simulink model "Blocos"  (R2022a)
settings: Solver=ode8  StartTime=0.0  StopTime=inf  FixedStep=0.01  RelTol=1e-3  EnableMultiTasking=on
libraries: dspstat3 x3
settings Model: Creator=MSI  LastModifiedBy=MSI
settings SolverCC: PositivePriorityOrder=on
settings OptimizationCC: EnhancedBackFolding=on  PassReuseOutputArgsAs=Individual arguments  ZeroExternalMemoryAtStartup=off  ZeroInternalMemoryAtStartup=off  MaxStackSize=64  OptimizeBlockOrder=speed  DifferentSizesBufferReuse=on  OptimizationCustomize=off  EfficientTunableParamExpr=on
settings DebuggingCC: ParameterTunabilityLossMsg=error
settings HardwareCC: ProdBitPerPointer=32  ProdBitPerSizeT=32  ProdBitPerPtrDiffT=32  ProdLargestAtomicInteger=Long  ProdLargestAtomicFloat=Double  ProdWordSize=32  ProdLongLongMode=on  ProdHWDeviceType=ARM Compatible->ARM Cortex
settings RTWCC: SystemTargetFile=ert.tlc  HardwareBoard=Raspberry Pi  TLCOptions="-aInlineSetEventsForThisBaseRateFcn=TLC_FALSE -aSuppressMultiTaskScheduler=TLC_FALSE  -aRateBasedStepFcn=0"  TemplateMakefile=ert_default_tmf  Toolchain=GNU GCC Embedded Linux  BuildConfiguration=Faster Runs
settings CodeAppCC: ForceParamTrailComments=on  IgnoreCustomStorageClasses=off  OperatorAnnotations=on  SimulinkDataObjDesc=on  SFDataObjDesc=on  InsertBlockDesc=on
settings ERTTargetCC: SupportVariableSizeSignals=on  ExtModeTransport=2  ExtModeStaticAlloc=on  ExtModeMexFile=ext_xcp  ExtModeIntrfLevel=Level2 - Open

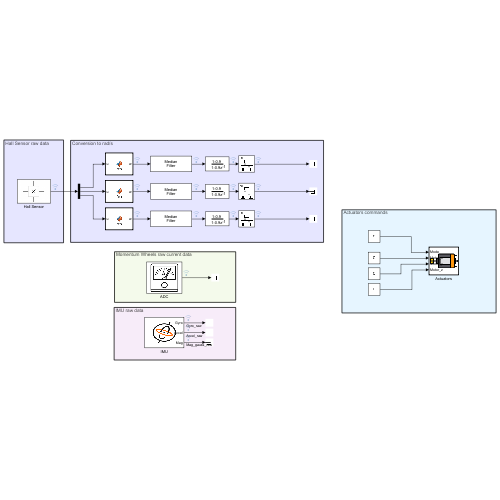
[thumbnail: Simulink's stored preview of the top-level diagram]
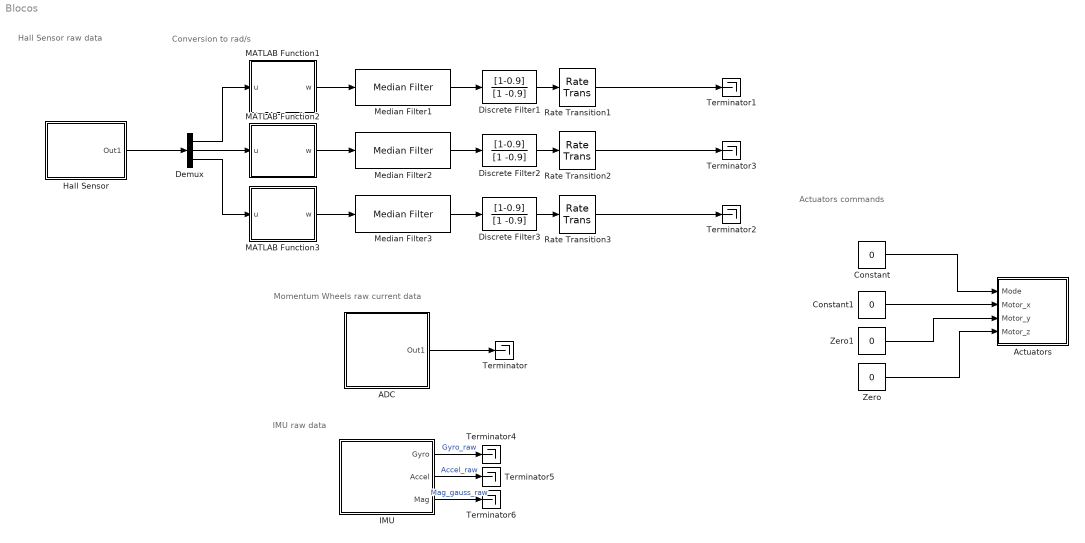
== system Blocos ==
  note: Actuators commands
  note: IMU raw data
  note: Momentum Wheels raw current data
  note: Hall Sensor raw data
  note: Conversion to rad/s
  ADC : Subsystem
      mask Display: image('$imagefile'); % Use "Edit Image" on toolstrip to change.
  Actuators : Subsystem  TreatAsAtomicUnit=on  SystemSampleTime=0.01
      mask Display: image('$imagefile'); % Use "Edit Image" on toolstrip to change.
  Constant : Constant  Value=0
  Constant1 : Constant  Value=0
  Demux : Demux  Outputs=3
  Discrete Filter1 : DiscreteFilter  Numerator=[1-0.9]  Denominator=[1 -0.9]  SampleTime=0.01
  Discrete Filter2 : DiscreteFilter  Numerator=[1-0.9]  Denominator=[1 -0.9]  SampleTime=0.01
  Discrete Filter3 : DiscreteFilter  Numerator=[1-0.9]  Denominator=[1 -0.9]  SampleTime=0.01
  Hall Sensor : Subsystem
      mask Display: image('$imagefile'); % Use "Edit Image" on toolstrip to change.
  IMU : Subsystem
      mask Display: image('$imagefile'); % Use "Edit Image" on toolstrip to change.
  MATLAB Function1 : MATLAB Function  TreatAsAtomicUnit=on
  MATLAB Function2 : MATLAB Function  TreatAsAtomicUnit=on
  MATLAB Function3 : MATLAB Function  TreatAsAtomicUnit=on
  Median Filter1 : dspstat3/Median Filter  WindowLength=5  SimulateUsing=Interpreted execution
      settings: SourceProductBaseCode=DS
  Median Filter2 : dspstat3/Median Filter  WindowLength=5  SimulateUsing=Interpreted execution
      settings: SourceProductBaseCode=DS
  Median Filter3 : dspstat3/Median Filter  WindowLength=5  SimulateUsing=Interpreted execution
      settings: SourceProductBaseCode=DS
  Rate Transition1 : RateTransition
  Rate Transition2 : RateTransition
  Rate Transition3 : RateTransition
  Terminator{,1..6} (7 alike) : Terminator
  Zero : Constant  Value=0  OutDataTypeStr=Inherit: Inherit via back propagation
  Zero1 : Constant  Value=0  OutDataTypeStr=Inherit: Inherit via back propagation
  wires:
  Constant/1 -> Actuators/1(Mode)
  Constant1/1 -> Actuators/2(Motor_x)
  Zero/1 -> Actuators/4(Motor_z)
  Zero1/1 -> Actuators/3(Motor_y)
  IMU/1(Gyro) -> Terminator4/1  "Gyro_raw"
  IMU/2(Accel) -> Terminator5/1  "Accel_raw"
  IMU/3(Mag) -> Terminator6/1  "Mag_gauss_raw"
  MATLAB Function3/1(w) -> Median Filter3/1
  MATLAB Function2/1(w) -> Median Filter2/1
  MATLAB Function1/1(w) -> Median Filter1/1
  Demux/2 -> MATLAB Function2/1(u)
  Demux/1 -> MATLAB Function1/1(u)
  Demux/3 -> MATLAB Function3/1(u)
  Discrete Filter3/1 -> Rate Transition3/1
  Rate Transition3/1 -> Terminator2/1
  Median Filter3/1 -> Discrete Filter3/1
  Rate Transition1/1 -> Terminator1/1
  Median Filter1/1 -> Discrete Filter1/1
  Discrete Filter1/1 -> Rate Transition1/1
  Rate Transition2/1 -> Terminator3/1
  Median Filter2/1 -> Discrete Filter2/1
  Discrete Filter2/1 -> Rate Transition2/1
  Hall Sensor/1(Out1) -> Demux/1
  ADC/1(Out1) -> Terminator/1

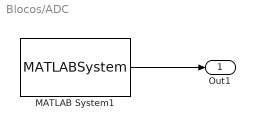
== system Blocos/ADC ==
  MATLAB System1 : MATLABSystem  System=read_current  SampleTime=0.01
      mask Type: read_current
      mask Display:
      | disp('ADC');
      | port_label('output',1,'current');
  Out1 : Outport
  wires:
  MATLAB System1/1 -> Out1/1

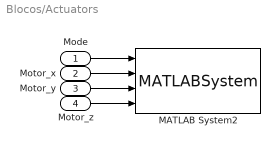
== system Blocos/Actuators ==
  Mode : Inport
  Motor_x : Inport  Port=2
  Motor_y : Inport  Port=3
  Motor_z : Inport  Port=4
  MATLAB System2 : MATLABSystem  System=arduinoPwmWrite
      mask Type: arduinoPwmWrite
      mask Display:
      | disp('PWM INO');
      | port_label('input',1,'mode');
      | port_label('input',2,'pwm_0');
      | port_label('input',3,'pwm_1');
      | port_label('input',4,'pwm_2');
  wires:
  Motor_y/1 -> MATLAB System2/3
  Motor_x/1 -> MATLAB System2/2
  Motor_z/1 -> MATLAB System2/4
  Mode/1 -> MATLAB System2/1

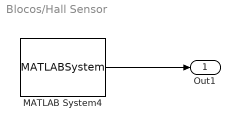
== system Blocos/Hall Sensor ==
  MATLAB System4 : MATLABSystem  System=read_n_crossings  SampleTime=0.01
      mask Type: read_n_crossings
      mask Display:
      | disp('Hall Sensor');
      | port_label('output',1,'n');
  Out1 : Outport
  wires:
  MATLAB System4/1 -> Out1/1

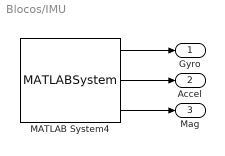
== system Blocos/IMU ==
  MATLAB System4 : MATLABSystem  System=read_imu  SampleTime=0.01
      mask Type: read_imu
      mask Display:
      | disp('IMU');
      | port_label('output',1,'gyro');
      | port_label('output',2,'accel');
      | port_label('output',3,'mag');
  Gyro : Outport
  Accel : Outport  Port=2
  Mag : Outport  Port=3
  wires:
  MATLAB System4/1 -> Gyro/1
  MATLAB System4/2 -> Accel/1
  MATLAB System4/3 -> Mag/1

== matlab function Blocos/MATLAB Function2 ==
  settings: updateMethod=DISCRETE  sampleTime=0.01
  data: u input; w output
function w = fcn(u)
    persistent counter;
    
    tw = 0.01;
    if isempty(counter) 
        counter = 0;
    end
        
    n = u-counter;
    counter = u;
    if (n~=0)
        w = n*pi/(4*tw);
    else
        w = 0;
    end

== matlab function Blocos/MATLAB Function3 ==
  settings: updateMethod=DISCRETE  sampleTime=0.01
  data: u input; w output
function w = fcn(u)
    persistent counter;
    
    tw = 0.01;
    if isempty(counter) 
        counter = 0;
    end
        
    n = u-counter;
    counter = u;
    if (n~=0)
        w = n*pi/(4*tw);
    else
        w = 0;
    end

== matlab function Blocos/MATLAB Function1 ==
  settings: updateMethod=DISCRETE  sampleTime=0.01
  data: u input; w output
function w = fcn(u)
    persistent counter;
    
    tw = 0.01;
    if isempty(counter) 
        counter = 0;
    end
        
    n = u-counter;
    counter = u;
    if (n~=0)
        w = n*pi/(4*tw);
    else
        w = 0;
    end
